simulink model "Example_8_2"  (R2014a)
settings: Solver=FixedStepDiscrete  StartTime=0.0  StopTime=10.0  FixedStep=1  RelTol=1e-3
libraries: dspsrcs4 x1
settings Model: Creator=Lee Edwards  LastModifiedBy=Lee
settings DataIOCC: SignalLoggingSaveFormat=ModelDataLogs
settings OptimizationCC: ExpressionDepthLimit=2147483647
settings DebuggingCC: UnderspecifiedInitializationDetection=Classic  FcnCallInpInsideContextMsg=UseLocalSettings  StateNameClashWarn=warning
settings GRTTargetCC: CombineOutputUpdateFcns=off  GRTInterface=on

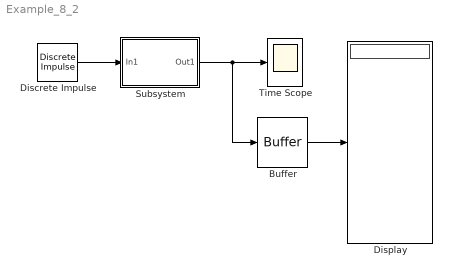
== system Example_8_2 ==
  Buffer : Buffer  N=10
  Discrete Impulse : dspsrcs4/Discrete  Impulse  Delay=0  SampleTime=1  FrameSample=1  dataType=double  isSigned=on  wordLen=16  udDataType=sfix(16)  fracBitsMode=Best precision  numFracBits=15  OutDataTypeStr=double  LastOutDataTypeStr=double
  Display : Display
  Subsystem : Subsystem
  Time Scope : Scope
      settings: DataFormat=Structure
  wires:
  Subsystem/1(Out1) -> Time Scope/1, Buffer/1
  Discrete Impulse/1 -> Subsystem/1(In1)
  Buffer/1 -> Display/1

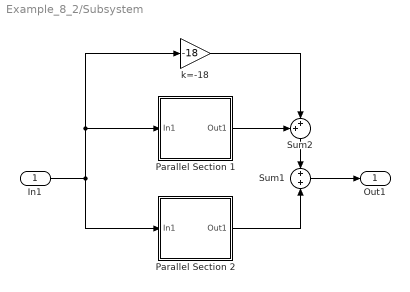
== system Example_8_2/Subsystem ==
  In1 : Inport
  Parallel Section 1 : Subsystem
  Parallel Section 2 : Subsystem
  Sum1 : Sum  Inputs=+|+
  Sum2 : Sum  Inputs=++|
  k=-18 : Gain  Gain=-18
  Out1 : Outport
  wires:
  In1/1 -> Parallel Section 1/1(In1), k=-18/1, Parallel Section 2/1(In1)
  Parallel Section 2/1(Out1) -> Sum1/2
  k=-18/1 -> Sum2/2
  Parallel Section 1/1(Out1) -> Sum2/1
  Sum2/1 -> Sum1/1
  Sum1/1 -> Out1/1

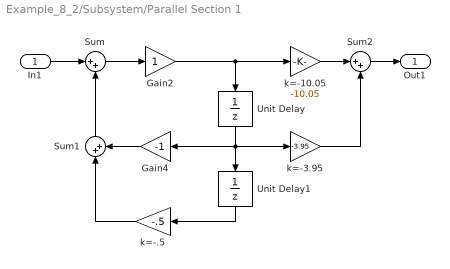
== system Example_8_2/Subsystem/Parallel Section 1 ==
  In1 : Inport
  Gain2 : Gain
  Gain4 : Gain  Gain=-1
  Sum : Sum  Inputs=|++
  Sum1 : Sum  Inputs=|++
  Sum2 : Sum  Inputs=|++
  Unit Delay : UnitDelay  SampleTime=-1
  Unit Delay1 : UnitDelay  SampleTime=-1
  k=-.5 : Gain  Gain=-.5
  k=-10.05 : Gain  Gain=-10.05
  k=-3.95 : Gain  Gain=-3.95
  Out1 : Outport
  wires:
  Unit Delay/1 -> Unit Delay1/1, Gain4/1, k=-3.95/1
  Unit Delay1/1 -> k=-.5/1
  In1/1 -> Sum/1
  Gain4/1 -> Sum1/2
  k=-.5/1 -> Sum1/1
  Sum1/1 -> Sum/2
  k=-3.95/1 -> Sum2/2
  Sum2/1 -> Out1/1
  Sum/1 -> Gain2/1
  Gain2/1 -> Unit Delay/1, k=-10.05/1
  k=-10.05/1 -> Sum2/1

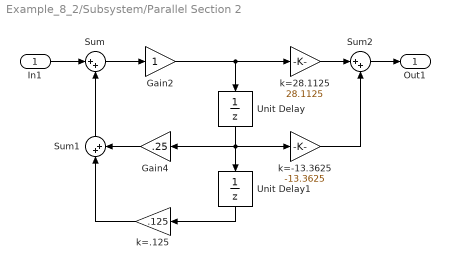
== system Example_8_2/Subsystem/Parallel Section 2 ==
  In1 : Inport
  Gain2 : Gain
  Gain4 : Gain  Gain=.25
  Sum : Sum  Inputs=|++
  Sum1 : Sum  Inputs=|++
  Sum2 : Sum  Inputs=|++
  Unit Delay : UnitDelay  SampleTime=-1
  Unit Delay1 : UnitDelay  SampleTime=-1
  k=-13.3625 : Gain  Gain=-13.3625
  k=.125 : Gain  Gain=.125
  k=28.1125 : Gain  Gain=28.1125
  Out1 : Outport
  wires:
  Unit Delay/1 -> Unit Delay1/1, Gain4/1, k=-13.3625/1
  Unit Delay1/1 -> k=.125/1
  In1/1 -> Sum/1
  Gain4/1 -> Sum1/2
  k=.125/1 -> Sum1/1
  Sum1/1 -> Sum/2
  k=-13.3625/1 -> Sum2/2
  Sum2/1 -> Out1/1
  Sum/1 -> Gain2/1
  Gain2/1 -> Unit Delay/1, k=28.1125/1
  k=28.1125/1 -> Sum2/1
